simulink model "DFIG_BESS_In_power_LFnetwork_5bus"  (R2017b)
settings: Solver=ode23tb  StartTime=0.0  StopTime=7.5  MaxStep=0.04  RelTol=1e-3  EnableMultiTasking=on
values from neighbouring files (symbols this model uses):
  beta = beta (k)    [Parameter_2M_DFIG_BESS.m]
  Cbus = 80e-3    (= 0.08)    [Parameter_2M_DFIG_BESS.m]
  Cbus_bess = 15e-3    (= 0.015)    [Parameter_2M_DFIG_BESS.m]
  Cfilter = 80e-3    (= 0.08)    [Parameter_2M_DFIG_BESS.m]
  cp_opt_abs = abs(max(Cp))    [Parameter_2M_DFIG_BESS.m]
  D = 0.1    [Parameter_2M_DFIG_BESS.m]
  f = 60    [Parameter_2M_DFIG_BESS.m]
  Fs = 1.5    [Parameter_2M_DFIG_BESS.m]
  fsw = 4e3    (= 4000)    [Parameter_2M_DFIG_BESS.m]
  J = 90    [Parameter_2M_DFIG_BESS.m]
  ki_id = (wni^2)*Lr*sigma    (= 491.599501999)    [Parameter_2M_DFIG_BESS.m]
  ki_idg = (wnig^2)*Lg    (= 68.6450725305)    [Parameter_2M_DFIG_BESS.m]
  ki_iq = ki_id    (= 491.599501999)    [Parameter_2M_DFIG_BESS.m]
  ki_iqg = ki_idg    (= 68.6450725305)    [Parameter_2M_DFIG_BESS.m]
  ki_v = -300000    [Parameter_2M_DFIG_BESS.m]
  kp_id = (2*wni*sigma*Lr)-Rr    (= 0.5771)    [Parameter_2M_DFIG_BESS.m]
  kp_idg = (2*wnig*Lg)-Rg    (= 0.364153420404)    [Parameter_2M_DFIG_BESS.m]
  kp_iq = kp_id    (= 0.5771)    [Parameter_2M_DFIG_BESS.m]
  kp_iqg = kp_idg    (= 0.364153420404)    [Parameter_2M_DFIG_BESS.m]
  kp_v = -1000    [Parameter_2M_DFIG_BESS.m]
  Kpg = 1/(1.5*Vs*sqrt(2/3))    [Parameter_2M_DFIG_BESS.m]
  Kqg = -Kpg    [Parameter_2M_DFIG_BESS.m]
  lambda_opt = abs(lambda(posicion))    [Parameter_2M_DFIG_BESS.m]
  Lfilter = 483e-6    (= 0.000483)    [Parameter_2M_DFIG_BESS.m]
  Lg = 483e-6    (= 0.000483)    [Parameter_2M_DFIG_BESS.m]
  Lm = 2.5e-3    (= 0.0025)    [Parameter_2M_DFIG_BESS.m]
  Lr = Lm + Lsr    (= 0.002587)    [Parameter_2M_DFIG_BESS.m]
  Ls = Lm + Lsi    (= 0.002587)    [Parameter_2M_DFIG_BESS.m]
  Lsi = 87e-6    (= 8.7e-05)    [Parameter_2M_DFIG_BESS.m]
  n = 1800    [Parameter_2M_DFIG_BESS.m]
  N = 100    [Parameter_2M_DFIG_BESS.m]
  p = 2    [Parameter_2M_DFIG_BESS.m]
  Ps = 2e6    (= 2000000)    [Parameter_2M_DFIG_BESS.m]
  Radio = 44    [Parameter_2M_DFIG_BESS.m]
  Rfilter = 20e-3    (= 0.02)    [Parameter_2M_DFIG_BESS.m]
  ro = 1.225    [Parameter_2M_DFIG_BESS.m]
  Rr = 2.9e-3    (= 0.0029)    [Parameter_2M_DFIG_BESS.m]
  Rs = 2.6e-3    (= 0.0026)    [Parameter_2M_DFIG_BESS.m]
  sigma = 1- Lm^2/(Ls*Lr)    (= 0.0661284179513)    [Parameter_2M_DFIG_BESS.m]
  Ts = 1/fsw/f    (= 4.16666666667e-06)    [Parameter_2M_DFIG_BESS.m]
  Vbus_ref = 1200    [Parameter_2M_DFIG_BESS.m]
  Vdc_bat_ref = 1300    [Parameter_2M_DFIG_BESS.m]
  Vs = 690    [Parameter_2M_DFIG_BESS.m]
undefined symbols (not defined in the file or in its folder): D1, D11, Delta, DiscIntNeverNeededParam, Ion, Lithium, sigbuilder_block
libraries: powerlib x83, powerlib_meascontrol x28, sps_avr x2, electricdrivelib x1, peGeneralControl x1
(part 2 of 3)

== system DFIG_BESS_In_power_LFnetwork_5bus/Load N°2 6MW 2Mvar ==
  note: Consumer Load
  3-Phase Breaker : powerlib/Elements/Three-Phase Breaker  Commented=on  InitialState=open  SwitchA=on  SwitchB=on  SwitchC=on  SwitchTimes=[7]  External=off  BreakerResistance=0.001  SnubberResistance=1e6  SnubberCapacitance=inf  Measurements=None
      settings: AttributesFormatString=\n
  Load : powerlib/Measurements/Three-Phase V-I Measurement  VoltageMeasurement=no  SetLabelV=on  LabelV=Vabc_Load_B3  Vpu=off  VpuLL=off  CurrentMeasurement=no  SetLabelI=on  LabelI=Iabc_Load_B3  Ipu=off  Pbase=25e3  Vbase=480  OutputType=Magnitude  PhasorSimulation=off  PSBequivalent=0
  Main Load 10MW : powerlib/Elements/Three-Phase Parallel RLC Load  LConnTagsString=A|B|C  Configuration=Y (grounded)  NominalVoltage=33e+03  Vabc=[1e3 1e3 1e3]  Vabcp=[1e3 1e3 1e3]  NominalFrequency=60  UnbalancedPower=off  ActivePower=6e+06  InductivePower=2e+06  CapacitivePower=0  Pabc=[10e3 9e3 11e3]  QLabc=[100 90 110]  QCabc=[100 90 110]  Pabcp=[10e3 9e3 11e3]  QLabcp=[100 90 110]  QCabcp=[100 90 110]  Measurements=None  LoadType=constant Z
  Main Load 10M : powerlib/Elements/Three-Phase Parallel RLC Load  Commented=on  LConnTagsString=A|B|C  Configuration=Y (grounded)  NominalVoltage=33e+03  Vabc=[1e3 1e3 1e3]  Vabcp=[1e3 1e3 1e3]  NominalFrequency=60  UnbalancedPower=off  ActivePower=10e+06  InductivePower=0  CapacitivePower=0  Pabc=[10e3 9e3 11e3]  QLabc=[100 90 110]  QCabc=[100 90 110]  Pabcp=[10e3 9e3 11e3]  QLabcp=[100 90 110]  QCabcp=[100 90 110]  Measurements=None  LoadType=constant Z
  PLL (3ph)1 : powerlib_meascontrol/PLL/PLL (3ph)  Commented=on  Fmin=45  Par_Init=[0, f]  ParK=[180, 3200, 1]  TcD=1e-4  MaxRateChangeFreq=12  FilterCutOffFreq=25  Ts=0  AGC=on
  "Power (3ph, Instantaneous)1" : powerlib_meascontrol/Measurements/Power (3ph, Instantaneous)  Commented=on
      settings: SourceProductName=Simscape Power Systems
  Scope : Scope  Commented=on
  Vbus vcc1 : From  Commented=on  GotoTag=Iabc_Load_B3  TagVisibility=global
  Vbus vcc2 : From  Commented=on  GotoTag=Vabc_Load_B3  TagVisibility=global
  A : PMIOPort  Port=1  Side=Right
  B : PMIOPort  Port=2  Side=Right
  C : PMIOPort  Port=3  Side=Right
  wires:
  Vbus vcc1/1 -> "Power (3ph, Instantaneous)1"/2
  Vbus vcc2/1 -> PLL (3ph)1/1, "Power (3ph, Instantaneous)1"/1
  "Power (3ph, Instantaneous)1"/1 -> Scope/1
  connections:
  3-Phase Breaker/LConn2 -- Load/RConn2 -- Main Load 10MW/LConn2
  3-Phase Breaker/LConn3 -- Load/RConn3 -- Main Load 10MW/LConn3
  3-Phase Breaker/LConn1 -- Load/RConn1 -- Main Load 10MW/LConn1
  3-Phase Breaker/RConn2 -- Main Load 10M/LConn2
  3-Phase Breaker/RConn1 -- Main Load 10M/LConn1
  3-Phase Breaker/RConn3 -- Main Load 10M/LConn3
  A/RConn1 -- Load/LConn1
  B/RConn1 -- Load/LConn2
  C/RConn1 -- Load/LConn3

== system DFIG_BESS_In_power_LFnetwork_5bus/Load N°3 24MW 5Mvar ==
  note: Consumer Load
  " Load" : powerlib/Elements/Three-Phase Parallel RLC Load  Commented=on  LConnTagsString=A|B|C  Configuration=Y (grounded)  NominalVoltage=33e+03  Vabc=[1e3 1e3 1e3]  Vabcp=[1e3 1e3 1e3]  NominalFrequency=60  UnbalancedPower=off  ActivePower=5e+06  InductivePower=0  CapacitivePower=0  Pabc=[10e3 9e3 11e3]  QLabc=[100 90 110]  QCabc=[100 90 110]  Pabcp=[10e3 9e3 11e3]  QLabcp=[100 90 110]  QCabcp=[100 90 110]  Measurements=None  LoadType=constant Z
  3-Phase Breaker : powerlib/Elements/Three-Phase Breaker  Commented=on  InitialState=open  SwitchA=on  SwitchB=on  SwitchC=on  SwitchTimes=[7]  External=off  BreakerResistance=0.001  SnubberResistance=1e6  SnubberCapacitance=inf  Measurements=None
      settings: AttributesFormatString=\n
  Load : powerlib/Measurements/Three-Phase V-I Measurement  VoltageMeasurement=no  SetLabelV=on  LabelV=Vabc_Load_B4  Vpu=off  VpuLL=off  CurrentMeasurement=no  SetLabelI=on  LabelI=Iabc_Load_B4  Ipu=off  Pbase=25e3  Vbase=480  OutputType=Magnitude  PhasorSimulation=off  PSBequivalent=0
  Main Load 10MW : powerlib/Elements/Three-Phase Parallel RLC Load  LConnTagsString=A|B|C  Configuration=Y (grounded)  NominalVoltage=33e+03  Vabc=[1e3 1e3 1e3]  Vabcp=[1e3 1e3 1e3]  NominalFrequency=60  UnbalancedPower=off  ActivePower=24e+06  InductivePower=5e+06  CapacitivePower=0  Pabc=[10e3 9e3 11e3]  QLabc=[100 90 110]  QCabc=[100 90 110]  Pabcp=[10e3 9e3 11e3]  QLabcp=[100 90 110]  QCabcp=[100 90 110]  Measurements=None  LoadType=constant Z
  PLL (3ph)1 : powerlib_meascontrol/PLL/PLL (3ph)  Commented=on  Fmin=45  Par_Init=[0, f]  ParK=[180, 3200, 1]  TcD=1e-4  MaxRateChangeFreq=12  FilterCutOffFreq=25  Ts=0  AGC=on
  "Power (3ph, Instantaneous)1" : powerlib_meascontrol/Measurements/Power (3ph, Instantaneous)  Commented=on
      settings: SourceProductName=Simscape Power Systems
  Scope : Scope  Commented=on
  Vbus vcc1 : From  Commented=on  GotoTag=Iabc_Load_B4  TagVisibility=global
  Vbus vcc2 : From  Commented=on  GotoTag=Vabc_Load_B4  TagVisibility=global
  A : PMIOPort  Port=1  Side=Right
  B : PMIOPort  Port=2  Side=Right
  C : PMIOPort  Port=3  Side=Right
  wires:
  "Power (3ph, Instantaneous)1"/1 -> Scope/1
  Vbus vcc2/1 -> "Power (3ph, Instantaneous)1"/1, PLL (3ph)1/1
  Vbus vcc1/1 -> "Power (3ph, Instantaneous)1"/2
  connections:
  C/RConn1 -- Load/LConn3
  B/RConn1 -- Load/LConn2
  A/RConn1 -- Load/LConn1
  3-Phase Breaker/RConn3 -- " Load"/LConn3
  3-Phase Breaker/RConn1 -- " Load"/LConn1
  3-Phase Breaker/RConn2 -- " Load"/LConn2
  Load/RConn1 -- 3-Phase Breaker/LConn1 -- Main Load 10MW/LConn1
  Load/RConn3 -- 3-Phase Breaker/LConn3 -- Main Load 10MW/LConn3
  Load/RConn2 -- 3-Phase Breaker/LConn2 -- Main Load 10MW/LConn2

== system DFIG_BESS_In_power_LFnetwork_5bus/Load N°4 12MW 3Mvar Load N°5 5MW 2Mvar ==
  note: Load 5
  note: Load 4
  " Load" : powerlib/Elements/Three-Phase Parallel RLC Load  Commented=on  LConnTagsString=A|B|C  Configuration=Y (grounded)  NominalVoltage=33e+03  Vabc=[1e3 1e3 1e3]  Vabcp=[1e3 1e3 1e3]  NominalFrequency=60  UnbalancedPower=off  ActivePower=5e+06  InductivePower=2e+06  CapacitivePower=0  Pabc=[10e3 9e3 11e3]  QLabc=[100 90 110]  QCabc=[100 90 110]  Pabcp=[10e3 9e3 11e3]  QLabcp=[100 90 110]  QCabcp=[100 90 110]  Measurements=None  LoadType=constant Z
  3-Phase Breaker : powerlib/Elements/Three-Phase Breaker  Commented=on  InitialState=open  SwitchA=on  SwitchB=on  SwitchC=on  SwitchTimes=[5]  External=off  BreakerResistance=0.001  SnubberResistance=1e6  SnubberCapacitance=inf  Measurements=None
      settings: AttributesFormatString=\n
  Load : powerlib/Measurements/Three-Phase V-I Measurement  VoltageMeasurement=no  SetLabelV=on  LabelV=Vabc_Load_B4  Vpu=off  VpuLL=off  CurrentMeasurement=no  SetLabelI=on  LabelI=Iabc_Load_B4  Ipu=off  Pbase=25e3  Vbase=480  OutputType=Magnitude  PhasorSimulation=off  PSBequivalent=0
  Main Load 10MW : powerlib/Elements/Three-Phase Parallel RLC Load  LConnTagsString=A|B|C  Configuration=Y (grounded)  NominalVoltage=33e+03  Vabc=[1e3 1e3 1e3]  Vabcp=[1e3 1e3 1e3]  NominalFrequency=60  UnbalancedPower=off  ActivePower=12e+06  InductivePower=3e+06  CapacitivePower=0  Pabc=[10e3 9e3 11e3]  QLabc=[100 90 110]  QCabc=[100 90 110]  Pabcp=[10e3 9e3 11e3]  QLabcp=[100 90 110]  QCabcp=[100 90 110]  Measurements=None  LoadType=constant Z
  PLL (3ph)1 : powerlib_meascontrol/PLL/PLL (3ph)  Commented=on  Fmin=45  Par_Init=[0, f]  ParK=[180, 3200, 1]  TcD=1e-4  MaxRateChangeFreq=12  FilterCutOffFreq=25  Ts=0  AGC=on
  "Power (3ph, Instantaneous)1" : powerlib_meascontrol/Measurements/Power (3ph, Instantaneous)  Commented=on
      settings: SourceProductName=Simscape Power Systems
  Scope : Scope  Commented=on
  Vbus vcc1 : From  Commented=on  GotoTag=Iabc_Load_B4  TagVisibility=global
  Vbus vcc2 : From  Commented=on  GotoTag=Vabc_Load_B4  TagVisibility=global
  A : PMIOPort  Port=1  Side=Right
  B : PMIOPort  Port=2  Side=Right
  C : PMIOPort  Port=3  Side=Right
  wires:
  Vbus vcc1/1 -> "Power (3ph, Instantaneous)1"/2
  Vbus vcc2/1 -> PLL (3ph)1/1, "Power (3ph, Instantaneous)1"/1
  "Power (3ph, Instantaneous)1"/1 -> Scope/1
  connections:
  Main Load 10MW/LConn2 -- 3-Phase Breaker/LConn2 -- Load/RConn2
  Main Load 10MW/LConn3 -- 3-Phase Breaker/LConn3 -- Load/RConn3
  Main Load 10MW/LConn1 -- 3-Phase Breaker/LConn1 -- Load/RConn1
  3-Phase Breaker/RConn2 -- " Load"/LConn2
  3-Phase Breaker/RConn1 -- " Load"/LConn1
  3-Phase Breaker/RConn3 -- " Load"/LConn3
  A/RConn1 -- Load/LConn1
  B/RConn1 -- Load/LConn2
  C/RConn1 -- Load/LConn3

== system DFIG_BESS_In_power_LFnetwork_5bus/Power ==
  "Power (3ph, Instantaneous)1" : powerlib_meascontrol/Measurements/Power (3ph, Instantaneous)
      settings: SourceProductName=Simscape Power Systems
  P : Outport
  wires:
  [Vabc_B1] -> "Power (3ph, Instantaneous)1"/1
  [Iabc_B1] -> "Power (3ph, Instantaneous)1"/2
  "Power (3ph, Instantaneous)1"/1 -> P/1

== system DFIG_BESS_In_power_LFnetwork_5bus/Power1 ==
  "Power (3ph, Instantaneous)1" : powerlib_meascontrol/Measurements/Power (3ph, Instantaneous)
      settings: SourceProductName=Simscape Power Systems
  P : Outport
  wires:
  "Power (3ph, Instantaneous)1"/1 -> P/1
  [Iabc_G] -> "Power (3ph, Instantaneous)1"/2
  [Vabc_G] -> "Power (3ph, Instantaneous)1"/1

== system DFIG_BESS_In_power_LFnetwork_5bus/Power2 ==
  "Power (3ph, Instantaneous)1" : powerlib_meascontrol/Measurements/Power (3ph, Instantaneous)
      settings: SourceProductName=Simscape Power Systems
  P : Outport
  wires:
  "Power (3ph, Instantaneous)1"/1 -> P/1
  [I_ac_g] -> "Power (3ph, Instantaneous)1"/2
  [V_ac_g] -> "Power (3ph, Instantaneous)1"/1

== system DFIG_BESS_In_power_LFnetwork_5bus/Power3 ==
  "Power (3ph, Instantaneous)1" : powerlib_meascontrol/Measurements/Power (3ph, Instantaneous)
      settings: SourceProductName=Simscape Power Systems
  P : Outport
  wires:
  [V_ac_bess_HV] -> "Power (3ph, Instantaneous)1"/1
  [I_ac_bess_HV] -> "Power (3ph, Instantaneous)1"/2
  "Power (3ph, Instantaneous)1"/1 -> P/1

== system DFIG_BESS_In_power_LFnetwork_5bus/Power4 ==
  "Power (3ph, Instantaneous)1" : powerlib_meascontrol/Measurements/Power (3ph, Instantaneous)
      settings: SourceProductName=Simscape Power Systems
  P : Outport
  wires:
  [V_ac_g_Total] -> "Power (3ph, Instantaneous)1"/1
  [I_ac_g_Total] -> "Power (3ph, Instantaneous)1"/2
  "Power (3ph, Instantaneous)1"/1 -> P/1

== system DFIG_BESS_In_power_LFnetwork_5bus/Subsystem1 ==
  " Iabc (pu)" : Scope  NumInputPorts=2
  " Load 3 MW 2 Mvar" : powerlib/Elements/Three-Phase Parallel RLC Load  LConnTagsString=A|B|C  Configuration=Y (grounded)  NominalVoltage=(13800)*0.98  Vabc=[1e3 1e3 1e3]  Vabcp=[1e3 1e3 1e3]  NominalFrequency=60  UnbalancedPower=off  ActivePower=3000000  InductivePower=2000000  CapacitivePower=0  Pabc=[10e3 9e3 11e3]  QLabc=[100 90 110]  QCabc=[100 90 110]  Pabcp=[10e3 9e3 11e3]  QLabcp=[100 90 110]  QCabcp=[100 90 110]  Measurements=None  LoadType=constant PQ
  " Speed (pu)" : Scope
  Bus Selector : BusSelector  OutputSignals="Stator current,Output active power   Peo (pu)"
  Bus Selector1 : BusSelector  OutputSignals="dq0 components.Stator voltage  vq (pu),dq0 components.Stator voltage  vd (pu),Mechanical.Rotor speed  wm  (pu),Mechanical.Rotor speed deviation  dw (pu),Output active power   Peo (pu)"
  Display3 : Display
  Excitation System : sps_avr/Excitation System  tr=20e-3  reg=[ 300, 0.001 ]  exc=[ 1, 0 ]  tgr=[ 0, 0 ]  damp=[ 0.001, 0.1 ]  sat=[ 0, 0 ]  lim=[ -11.5, 11.5, 0 ]  v0=[1,1.29071]
      settings: SourceProductName=Simscape Power Systems  SourceProductBaseCode=PS
  Ground : Ground
  HTG : powerlib/Machines/Hydraulic Turbine and Governor  sm="[ 10/3  0.07 ]"  gate="[  0.01  0.97518  -0.1  0.1 ]"  reg="[  0.05  1.163  0.105  0  0.01  ]"  hyd="[  0  2.67  ]"  dref=0  po=1
      settings: SourceProductName=Simscape Power Systems  SourceProductBaseCode=PS
  Pref : Constant
  "Synchronous Machine " : powerlib/Machines/Synchronous Machine pu Standard  PresetModel=No  MechanicalLoad=Mechanical power Pm  ShowDetailedParameters=on  RotorType=Salient-pole  Units=per unit standard parameters  MeasurementBus=off  NominalParameters="[50e+06  13800   f ]"  Reactances1=[ 31 32 33 34 35 36 37 ]  Reactances2=[ 1.305, 0.296, 0.252, 0.474, 0.243, 0.18 ]  dAxisTimeConstants=Short-circuit  qAxisTimeConstants=Open-circuit  TimeConstants1=[]  TimeConstants2=[]  TimeConstants3=[]  TimeConstants4=[]  TimeConstants5=[ 1.01, 0.053, 0.1 ]  TimeConstants6=[]  TimeConstants7=[]  TimeConstants8=[]  StatorResistance=2.8544e-3  Mechanical=[ 3.2 0 2]  PolePairs=2  InitialConditions=[0 -94.2826 0.750185 0.750185 0.750185 -24.943 -144.943 95.057 1.29071]  SetSaturation=off  Saturation=[0.6404,0.7127,0.8441,0.9214,0.9956,1.082,1.19,1.316,1.457;0.7,0.7698,0.8872,0.9466,0.9969,1.046,1.1,1.151,1.201]  LoadFlowParameters=[1 150000000 0 0]  TsPowergui=0  TsBlock=-1  IterativeModel=Trapezoidal non iterative  IterativeDiscreteModel=Trapezoidal non iterative  BusType=PQ  Pref=50e+06  Qref=0  Qmin=-Inf  Qmax=Inf  PLF=0  QLF=0
      settings: AttributesFormatString=\n\n  SourceProductName=Simscape Power Systems
  Terminator5 : Terminator
  Vf (pu) : Scope
  Vref : Constant
  wref : Constant
  Va : PMIOPort  Port=1  Side=Left
  Vb : PMIOPort  Port=2  Side=Left
  Vc : PMIOPort  Port=3  Side=Left
  wires:
  HTG/1 -> Display3/1, "Synchronous Machine "/1
  Bus Selector/2 -> " Iabc (pu)"/2  "<Output active power   Peo (pu)>"
  "Synchronous Machine "/1 -> Bus Selector1/1, Bus Selector/1
  Vref/1 -> Excitation System/1
  wref/1 -> HTG/1
  Pref/1 -> HTG/2
  Bus Selector1/4 -> HTG/5  "<Rotor speed deviation  dw (pu)>"
  Excitation System/1 -> "Synchronous Machine "/2, Vf (pu)/1
  Bus Selector1/1 -> Excitation System/3  "<Stator voltage  vq (pu)>"
  Ground/1 -> Excitation System/4
  Bus Selector1/2 -> Excitation System/2  "<Stator voltage  vd (pu)>"
  Bus Selector/1 -> " Iabc (pu)"/1  "<Stator current>"
  Bus Selector1/3 -> " Speed (pu)"/1, HTG/3  "<Rotor speed  wm  (pu)>"
  HTG/2 -> Terminator5/1
  Bus Selector1/5 -> HTG/4  "<Output active power   Peo (pu)>"
  connections:
  " Load 3 MW 2 Mvar"/LConn3 -- "Synchronous Machine "/RConn3 -- Vc/RConn1
  " Load 3 MW 2 Mvar"/LConn2 -- Vb/RConn1 -- "Synchronous Machine "/RConn2
  " Load 3 MW 2 Mvar"/LConn1 -- "Synchronous Machine "/RConn1 -- Va/RConn1

== system DFIG_BESS_In_power_LFnetwork_5bus/Subsystem2 ==
  " Iabc (pu)" : Scope  NumInputPorts=2
  " Load 3 MW 2 Mvar" : powerlib/Elements/Three-Phase Parallel RLC Load  LConnTagsString=A|B|C  Configuration=Y (grounded)  NominalVoltage=(13800)*0.98  Vabc=[1e3 1e3 1e3]  Vabcp=[1e3 1e3 1e3]  NominalFrequency=60  UnbalancedPower=off  ActivePower=3000000  InductivePower=2000000  CapacitivePower=0  Pabc=[10e3 9e3 11e3]  QLabc=[100 90 110]  QCabc=[100 90 110]  Pabcp=[10e3 9e3 11e3]  QLabcp=[100 90 110]  QCabcp=[100 90 110]  Measurements=None  LoadType=constant PQ
  " Speed (pu)" : Scope
  Bus Selector : BusSelector  OutputSignals="Stator current,Output active power   Peo (pu)"
  Bus Selector1 : BusSelector  OutputSignals="dq0 components.Stator voltage  vq (pu),dq0 components.Stator voltage  vd (pu),Mechanical.Rotor speed  wm  (pu),Mechanical.Rotor speed deviation  dw (pu),Output active power   Peo (pu)"
  Display3 : Display
  Excitation System : sps_avr/Excitation System  tr=20e-3  reg=[ 300, 0.001 ]  exc=[ 1, 0 ]  tgr=[ 0, 0 ]  damp=[ 0.001, 0.1 ]  sat=[ 0, 0 ]  lim=[ -11.5, 11.5, 0 ]  v0=[1,1.29071]
      settings: SourceProductName=Simscape Power Systems  SourceProductBaseCode=PS
  Ground : Ground
  HTG : powerlib/Machines/Hydraulic Turbine and Governor  sm="[ 10/3  0.07 ]"  gate="[  0.01  0.97518  -0.1  0.1 ]"  reg="[  0.05  1.163  0.105  0  0.01  ]"  hyd="[  0  2.67  ]"  dref=0  po=1
      settings: SourceProductName=Simscape Power Systems  SourceProductBaseCode=PS
  Pref : Constant
  "Synchronous Machine " : powerlib/Machines/Synchronous Machine pu Standard  PresetModel=No  MechanicalLoad=Mechanical power Pm  ShowDetailedParameters=on  RotorType=Salient-pole  Units=per unit standard parameters  MeasurementBus=off  NominalParameters="[30e+06  13800   f ]"  Reactances1=[ 31 32 33 34 35 36 37 ]  Reactances2=[ 1.305, 0.296, 0.252, 0.474, 0.243, 0.18 ]  dAxisTimeConstants=Short-circuit  qAxisTimeConstants=Open-circuit  TimeConstants1=[]  TimeConstants2=[]  TimeConstants3=[]  TimeConstants4=[]  TimeConstants5=[ 1.01, 0.053, 0.1 ]  TimeConstants6=[]  TimeConstants7=[]  TimeConstants8=[]  StatorResistance=2.8544e-3  Mechanical=[ 3.2 0 2]  PolePairs=2  InitialConditions=[0 -94.2826 0.750185 0.750185 0.750185 -24.943 -144.943 95.057 1.29071]  SetSaturation=off  Saturation=[0.6404,0.7127,0.8441,0.9214,0.9956,1.082,1.19,1.316,1.457;0.7,0.7698,0.8872,0.9466,0.9969,1.046,1.1,1.151,1.201]  LoadFlowParameters=[1 150000000 0 0]  TsPowergui=0  TsBlock=-1  IterativeModel=Trapezoidal non iterative  IterativeDiscreteModel=Trapezoidal non iterative  BusType=PQ  Pref=30e+06  Qref=0  Qmin=-Inf  Qmax=Inf  PLF=0  QLF=0
      settings: AttributesFormatString=\n\n  SourceProductName=Simscape Power Systems
  Terminator5 : Terminator
  Vf (pu) : Scope
  Vref : Constant
  wref : Constant
  Va : PMIOPort  Port=1  Side=Left
  Vb : PMIOPort  Port=2  Side=Left
  Vc : PMIOPort  Port=3  Side=Left
  wires:
  Bus Selector1/5 -> HTG/4  "<Output active power   Peo (pu)>"
  HTG/2 -> Terminator5/1
  Bus Selector1/3 -> HTG/3, " Speed (pu)"/1  "<Rotor speed  wm  (pu)>"
  Bus Selector/1 -> " Iabc (pu)"/1  "<Stator current>"
  Bus Selector1/2 -> Excitation System/2  "<Stator voltage  vd (pu)>"
  Ground/1 -> Excitation System/4
  Bus Selector1/1 -> Excitation System/3  "<Stator voltage  vq (pu)>"
  Excitation System/1 -> Vf (pu)/1, "Synchronous Machine "/2
  Bus Selector1/4 -> HTG/5  "<Rotor speed deviation  dw (pu)>"
  Pref/1 -> HTG/2
  wref/1 -> HTG/1
  Vref/1 -> Excitation System/1
  "Synchronous Machine "/1 -> Bus Selector/1, Bus Selector1/1
  Bus Selector/2 -> " Iabc (pu)"/2  "<Output active power   Peo (pu)>"
  HTG/1 -> "Synchronous Machine "/1, Display3/1
  connections:
  "Synchronous Machine "/RConn1 -- " Load 3 MW 2 Mvar"/LConn1 -- Va/RConn1
  Vb/RConn1 -- " Load 3 MW 2 Mvar"/LConn2 -- "Synchronous Machine "/RConn2
  "Synchronous Machine "/RConn3 -- " Load 3 MW 2 Mvar"/LConn3 -- Vc/RConn1

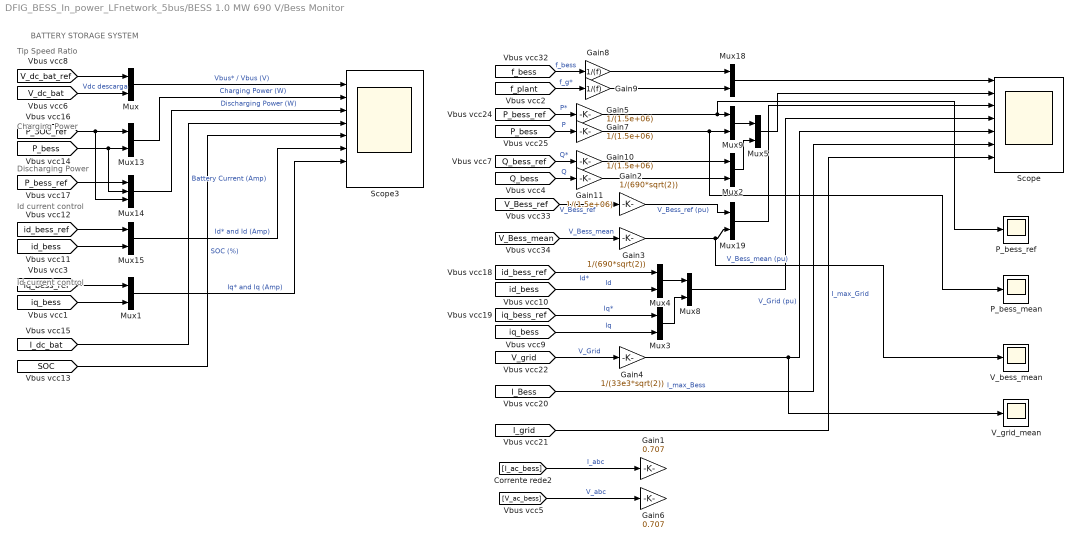
== system DFIG_BESS_In_power_LFnetwork_5bus/BESS 1.0 MW 690 V/Bess Monitor ==
  note: BATTERY STORAGE SYSTEM
  note: Tip Speed Ratio
  note: Charging Power
  note: Discharging Power
  note: Id current control
  note: Id current control
  Gain1 : Gain  Gain=0.707
  Gain{5,7,10..11} (4 alike) : Gain  Gain=1/(1.5e+06)
  Gain2 : Gain  Gain=1/(690*sqrt(2))
  Gain3 : Gain  Gain=1/(690*sqrt(2))
  Gain4 : Gain  Gain=1/(33e3*sqrt(2))
  Gain6 : Gain  Gain=0.707
  Gain8 : Gain  Gain=1/(f)
  Gain9 : Gain  Gain=1/(f)
  Mux{,1..5,8..9,13,15,18..19} (12 alike) : Mux  Inputs=2
  Mux14 : Mux  Inputs=3
  P_bess_mean : Scope
  P_bess_ref : Scope
  Scope : Scope  NumInputPorts=8
  Scope3 : Scope  NumInputPorts=8
  V_bess_mean : Scope
  V_grid_mean : Scope
  wires:
  [P_bess_ref] -> Mux14/1
  Mux13/1 -> Scope3/2  "Charging Power (W)"
  [P_SOC_ref] -> Mux14/3, Mux13/1
  [P_bess] -> Mux14/2, Mux13/2
  [id_bess_ref] -> Mux15/1
  [V_dc_bat_ref] -> Mux/1
  Mux/1 -> Scope3/1  "Vbus* / Vbus (V)"
  [id_bess] -> Mux15/2
  Mux14/1 -> Scope3/3  "Discharging Power (W)"
  [SOC] -> Scope3/5  "SOC (%)"
  [I_dc_bat] -> Scope3/4  "Battery Current (Amp)"
  Mux15/1 -> Scope3/6  "Id* and Id (Amp)"
  [V_dc_bat] -> Mux/2  "Vdc descarga"
  [iq_bess] -> Mux1/2
  [iq_bess_ref] -> Mux1/1
  Mux1/1 -> Scope3/7  "Iq* and Iq (Amp)"
  [Q_bess_ref] -> Gain10/1  "Q*"
  [iq_bess_ref] -> Mux3/1  "Iq*"
  [id_bess] -> Mux4/2  "Id"
  [iq_bess] -> Mux3/2  "Iq"
  [id_bess_ref] -> Mux4/1  "Id*"
  Mux4/1 -> Mux8/1
  Mux3/1 -> Mux8/2
  [P_bess_ref] -> Gain5/1  "P*"
  [f_bess] -> Gain8/1  "f_bess"
  [f_plant] -> Gain9/1  "f_g*"
  Mux18/1 -> Scope/1
  [V_Bess_ref] -> Gain2/1  "V_Bess_ref"
  [V_Bess_mean] -> Gain3/1  "V_Bess_mean"
  [V_ac_bess] -> Gain6/1  "V_abc"
  [I_ac_bess] -> Gain1/1  "I_abc"
  [V_grid] -> Gain4/1  "V_Grid"
  [P_bess] -> Gain7/1  "P"
  [Q_bess] -> Gain11/1  "Q"
  Gain2/1 -> Mux19/1  "V_Bess_ref (pu)"
  Gain3/1 -> V_bess_mean/1, Mux19/2  "V_Bess_mean (pu)"
  Gain4/1 -> V_grid_mean/1, Scope/5  "V_Grid (pu)"
  [I_Bess] -> Scope/6  "I_max_Bess"
  [I_grid] -> Scope/7  "I_max_Grid"
  Mux19/1 -> Scope/3
  Mux8/1 -> Scope/4
  Gain5/1 -> P_bess_ref/1, Mux9/1
  Gain7/1 -> P_bess_mean/1, Mux9/2
  Gain8/1 -> Mux18/1
  Gain9/1 -> Mux18/2
  Mux9/1 -> Mux5/1
  Mux2/1 -> Mux5/2
  Mux5/1 -> Scope/2
  Gain10/1 -> Mux2/1
  Gain11/1 -> Mux2/2

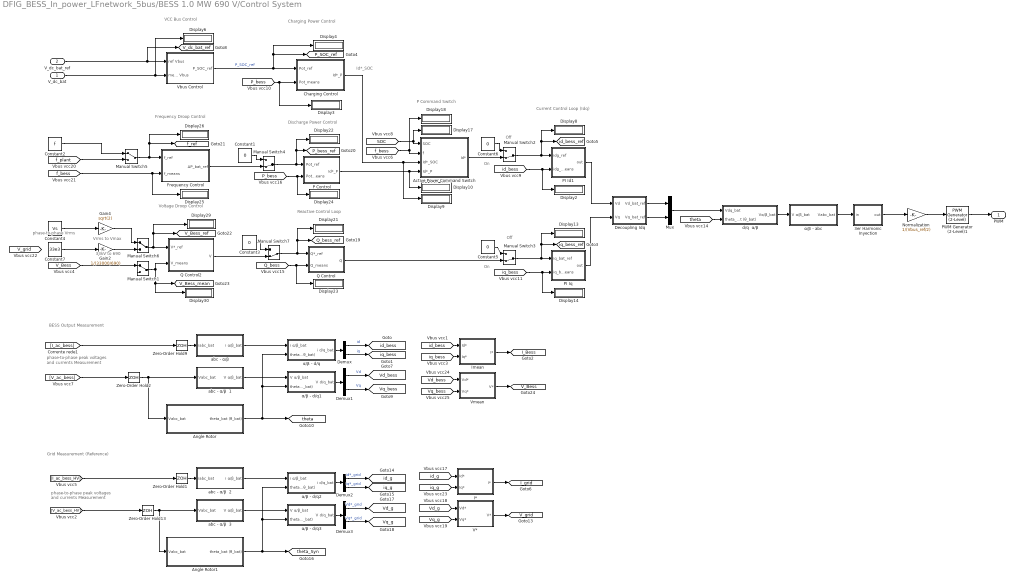
== system DFIG_BESS_In_power_LFnetwork_5bus/BESS 1.0 MW 690 V/Control System ==
  note: BESS Output Measurement
  note: Id*_SOC
  note: Grid Measurement (Reference)
  note: Current Control Loop (Idq)
  note: Discharge Power Control
  note: Frequency Droop Control
  note: VCC Bus Control
  note: Charging Power Control
  note: P Command Switch
  note: On
  note: Off
  note: On
  note: Off
  note: phase-to-phase peak voltages
      | and currents Measurement
  note: phase-to-phase peak voltages
      | and currents Measurement
  note: 33kV to 690
  note: Voltage Droop Control
  note: Reactive Control Loop
  note: Vrms to Vmax
  note: phase-to-phase Vrms
  V_dc_bat : Inport
  V_dc_bat_ref : Inport  Port=2
  " Angle Rotor" : Subsystem
  " Angle Rotor1" : Subsystem
  3er Harmonic Inyection : Subsystem
  Active Power Command Switch : Subsystem
  Charging Control : Subsystem
  Constant{1,3,5..6} (4 alike) : Constant  Value=0
  Constant2 : Constant  Value=f
  Constant4 : Constant  Value=Vs
  Constant7 : Constant  Value=33e3
  Decoupling Idq : Subsystem
  Demux{,1..3} (4 alike) : Demux  Outputs=2
  Display{2..4,6,8..10,13..14,17..18,21..26,29..30} (19 alike) : Display
  Frequency Control : Subsystem
  Gain2 : Gain  Gain=1/(33000/690)
  Gain4 : Gain  Gain=sqrt(2)
  I* : Subsystem
  Imean : Subsystem
  Manual Switch1 : ManualSwitch
  Manual Switch{2..4,7} (4 alike) : ManualSwitch  CurrentSetting=0
  Manual Switch5 : ManualSwitch
  Manual Switch6 : ManualSwitch
  Mux : Mux  Inputs=2
  Normalization : Gain  Gain=1/(Vbus_ref/2)
  P Control : Subsystem
  PI Id1 : Subsystem
  PI Iq : Subsystem
  PWM Generator (2-Level)1 : powerlib_meascontrol/Pulse & Signal Generators/PWM Generator (2-Level)  ModulatorType=Three-phase bridge (6 pulses)  ModulatorMode=Unsynchronized  Fc=fsw  Pc=0  nF=27  MinMax="[ -1  1 ]"  SamplingTechnique=Natural  ModulatingSignals=off  m=0.8  Freq=60  Phase=0  Ts=0  ShowCarrierOutport=off
      settings: SourceProductName=Simscape Power Systems
  Q Control : Subsystem
  Q Control2 : Subsystem
  V* : Subsystem
  Vbus Control : Subsystem
  Vmean : Subsystem
  Zero-Order Hold{1..2,9,13} (4 alike) : ZeroOrderHold  SampleTime=1/fsw
  "abc - α/β  " : Subsystem
  abc - α/β  1 : Subsystem
  abc - α/β  2 : Subsystem
  abc - α/β  3 : Subsystem
  "d/q  α/β " : Subsystem
  α/β - abc : Subsystem
  α/β - d/q : Subsystem
  α/β - d/q1 : Subsystem
  α/β - d/q2 : Subsystem
  α/β - d/q3 : Subsystem
  PWM : Outport
  tag scope: I_Bess=global, I_grid=global, P_SOC_ref=global, P_bess_ref=global, Q_bess_ref=global, V_Bess=global, V_Bess_mean=global, V_Bess_ref=global, V_dc_bat_ref=global, V_grid=global, Vd_bess=global, Vd_g=global, Vq_bess=global, Vq_g=global, f_ref=global, id_bess=global, id_bess_ref=global, id_g=global, iq_bess=global, iq_bess_ref=global, iq_g=global, theta=global, theta_Syn=global
  wires:
  PWM Generator (2-Level)1/1 -> PWM/1
  α/β - d/q/1(i d/q_bat) -> Demux/1
  Zero-Order Hold2/1 -> " Angle Rotor"/1(Vabc_bat), abc - α/β  1/1(Vabc_bat)
  α/β - abc/1(Vabc_bat) -> 3er Harmonic Inyection/1(in)
  Zero-Order Hold9/1 -> "abc - α/β  "/1(iabc_bat)
  "d/q  α/β "/1("Vα/β_bat ") -> α/β - abc/1(V α/β_bat)
  "abc - α/β  "/1(i α/β_bat) -> α/β - d/q/1(i α/β_bat)
  3er Harmonic Inyection/1(out) -> Normalization/1
  PI Id1/1(out) -> Decoupling Idq/1(Vd)
  PI Iq/1("out ") -> Decoupling Idq/2(Vq)
  Normalization/1 -> PWM Generator (2-Level)1/1
  V_dc_bat/1 -> Display6/1, Vbus Control/2("means Vbus ")
  [f_bess] -> Active Power Command Switch/2(f), Display18/1
  [SOC] -> Active Power Command Switch/1(SOC), Display17/1
  V_dc_bat_ref/1 -> [V_dc_bat_ref], Vbus Control/1("ref Vbus ")
  Vbus Control/1(P_SOC_ref) -> [P_SOC_ref], Display4/1, Charging Control/1("Pot_ref ")  "P_SOC_ref"
  [P_bess] -> Charging Control/2("Pot_means "), Display3/1
  Demux1/1 -> [Vd_bess]  "Vd"
  abc - α/β  1/1(V α/β_bat) -> α/β - d/q1/1(V α/β_bat)
  α/β - d/q1/1(V d/q_bat) -> Demux1/1
  Demux1/2 -> [Vq_bess]  "Vq"
  Mux/1 -> "d/q  α/β "/1(Vdq_bat)
  Decoupling Idq/1(" Vd_bat_ref") -> Mux/1
  Decoupling Idq/2(" Vq_bat_ref") -> Mux/2
  " Angle Rotor"/1(theta_bat (θ_bat)) -> α/β - d/q1/2(theta_bat (θ_bat)), α/β - d/q/2(theta_bat (θ_bat)), [theta]
  Demux/1 -> [id_bess]  "id"
  Demux/2 -> [iq_bess]  "iq"
  [theta] -> "d/q  α/β "/2(theta_bat (θ_bat))
  [id_bess] -> PI Id1/2(idg_means), Display2/1
  [iq_bess] -> Display14/1, PI Iq/2(iq_bat_means)
  Demux3/2 -> [Vq_g]  "Vq*_grid"
  Demux3/1 -> [Vd_g]  "Vd*_grid"
  abc - α/β  3/1(V α/β_bat) -> α/β - d/q3/1(V α/β_bat)
  abc - α/β  2/1(i α/β_bat) -> α/β - d/q2/1(i α/β_bat)
  " Angle Rotor1"/1(theta_bat (θ_bat)) -> α/β - d/q3/2(theta_bat (θ_bat)), α/β - d/q2/2(theta_bat (θ_bat)), [theta_Syn]
  Demux2/1 -> [id_g]  "id*_grid"
  Demux2/2 -> [iq_g]  "iq*_grid"
  α/β - d/q2/1(i d/q_bat) -> Demux2/1
  α/β - d/q3/1(V d/q_bat) -> Demux3/1
  [I_ac_bess_HV] -> Zero-Order Hold1/1
  [V_ac_bess_HV] -> Zero-Order Hold13/1
  Zero-Order Hold1/1 -> abc - α/β  2/1(iabc_bat)
  Zero-Order Hold13/1 -> " Angle Rotor1"/1(Vabc_bat), abc - α/β  3/1(Vabc_bat)
  [P_bess] -> Display24/1, P Control/2("Pot_means ")
  Manual Switch2/1 -> Display8/1, [id_bess_ref], PI Id1/1(idg_ref)
  Manual Switch3/1 -> Display13/1, [iq_bess_ref], PI Iq/1(iq_bat_ref)
  [f_bess] -> Display25/1, Frequency Control/2(f_means)
  Manual Switch4/1 -> [P_bess_ref], Display22/1, P Control/1("Pot_ref ")
  Frequency Control/1("ΔP_bat_ref ") -> Manual Switch4/2
  Constant1/1 -> Manual Switch4/1
  Manual Switch5/1 -> Display26/1, [f_ref], Frequency Control/1(f_ref)
  [Vq_g] -> V*/2(Vq*)
  [Vd_g] -> V*/1(Vd*)
  [Vd_bess] -> Vmean/1(Vd*)
  [Vq_bess] -> Vmean/2(Vq*)
  [f_plant] -> Manual Switch5/2
  Constant2/1 -> Manual Switch5/1
  Constant5/1 -> Manual Switch3/1
  V*/1("V* ") -> [V_grid]
  Vmean/1("V* ") -> [V_Bess]
  [I_ac_bess] -> Zero-Order Hold9/1
  [V_ac_bess] -> Zero-Order Hold2/1
  Active Power Command Switch/1(Id*) -> Manual Switch2/2
  Charging Control/1(Id*_P) -> Display9/1, Active Power Command Switch/3(Id*_SOC)
  P Control/1(Id*_P) -> Active Power Command Switch/4(Id*_P), Display10/1
  Imean/1("I* ") -> [I_Bess]
  [iq_bess] -> Imean/2(Iq*)
  [id_bess] -> Imean/1(Id*)
  I*/1("I* ") -> [I_grid]
  [id_g] -> I*/1(Id*)
  [iq_g] -> I*/2(Iq*)
  Constant6/1 -> Manual Switch2/1
  [V_Bess] -> Manual Switch1/1
  Manual Switch1/1 -> Q Control2/2(V_means), Display30/1, [V_Bess_mean]
  Q Control/1("Q ") -> Manual Switch3/2
  Constant3/1 -> Manual Switch7/1
  Gain4/1 -> Manual Switch6/1
  Constant4/1 -> Gain4/1
  Manual Switch7/1 -> [Q_bess_ref], Display21/1, Q Control/1(Q*_ref)
  Q Control2/1("V ") -> Manual Switch7/2
  Gain2/1 -> Manual Switch6/2
  Manual Switch6/1 -> Q Control2/1(V*_ref), Display29/1, [V_Bess_ref]
  [Q_bess] -> Display23/1, Q Control/2(Q_means)
  Constant7/1 -> Gain2/1

== system DFIG_BESS_In_power_LFnetwork_5bus/BESS 1.0 MW 690 V/Measurement of Power - Frequency ==
  FP : Fcn  Commented=on  Expr=cos(atan(u[1]/u[2]))
  Manual Switch3 : ManualSwitch  CurrentSetting=0
  Mux : Mux  Commented=on  Inputs=2
  PLL (3ph)1 : powerlib_meascontrol/PLL/PLL (3ph)  Fmin=45  Par_Init=[0, f]  ParK=[180, 3200, 1]  TcD=1e-4  MaxRateChangeFreq=12  FilterCutOffFreq=25  Ts=0  AGC=on
  "Power (3ph, Instantaneous)1" : powerlib_meascontrol/Measurements/Power (3ph, Instantaneous)
      settings: SourceProductName=Simscape Power Systems
  Scope : Scope  Commented=on
  F (Hz) : Outport
  P (W) : Outport  Port=2
  Q (VAR) : Outport  Port=3
  Angle (0) : Outport  Port=4
  tag scope: P_bess=global, Q_bess=global, f_bess=global, wt_mean=global
  wires:
  [V_ac_bess] -> "Power (3ph, Instantaneous)1"/1, PLL (3ph)1/1
  "Power (3ph, Instantaneous)1"/1 -> [P_bess], Mux/2, P (W)/1  "Pot"
  [I_ac_bess] -> "Power (3ph, Instantaneous)1"/2
  "Power (3ph, Instantaneous)1"/2 -> Mux/1, Q (VAR)/1, [Q_bess]
  PLL (3ph)1/2 -> Angle (0)/1, [wt_mean]
  Mux/1 -> FP/1
  FP/1 -> Scope/1
  [f_dfig_bess] -> Manual Switch3/1
  PLL (3ph)1/1 -> Manual Switch3/2
  Manual Switch3/1 -> F (Hz)/1, [f_bess]

== system DFIG_BESS_In_power_LFnetwork_5bus/BESS 1.0 MW 690 V/Subsystem1 ==
  In1 : Inport
  Bus Selector : BusSelector  OutputSignals=SOC (%),Current (A),Voltage (V)
  tag scope: I_dc_bat=global, SOC=global, V_dc_bat=global
  wires:
  Bus Selector/3 -> [V_dc_bat]  "<Voltage (V)>"
  Bus Selector/1 -> [SOC]  "<SOC (%)>"
  In1/1 -> Bus Selector/1
  Bus Selector/2 -> [I_dc_bat]  "<Current (A)>"

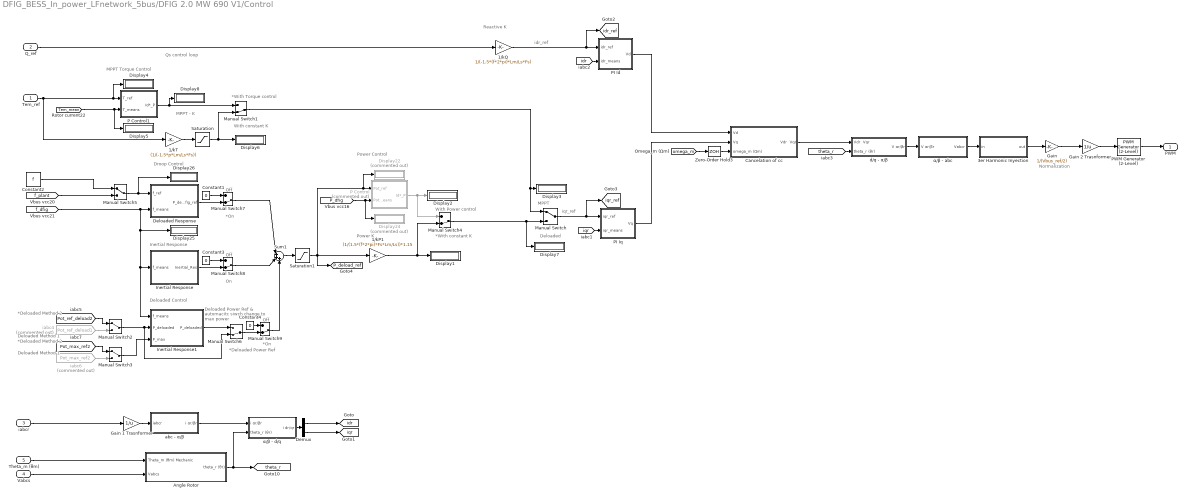
== system DFIG_BESS_In_power_LFnetwork_5bus/DFIG 2.0 MW 690 V1/Control ==
  note: Normalization
  note: iqr_ref
  note: idr_ref
  note: Qs control loop
  note: Reactive K
  note: MPPT - K
  note: Droop Control
  note: Power Control
  note: Power K
  note: MPPT
  note: Deloaded
  note: MPPT Torque Control
  note: Inertial Response
  note: Deloaded Control
  note: *Deloaded Power Ref
  note: Deloaded Power Ref &
      | automacitc siwch change
      | to max power
  note: *With constant K
  note: With Power control
  note: *With Torque control
  note: With constant K
  note: Deloaded Method 1
  note: Deloaded Method 1
  note: *Deloaded Method 2
  note: *Deloaded Method 2
  note: On
  note: *On
  note: *On
  note: Off
  note: Off
  note: Off
  Tem_ref : Inport
  Q_ref : Inport  Port=2
  iabcr : Inport  Port=3
  Vabcs : Inport  Port=4
  Theta_m (θm) : Inport  Port=5
  " Angle Rotor" : Subsystem
  1/kP1 : Gain  Gain=(1/(1.5*(f*2*pi)*Fs*Lm/Ls))*1.15
  1/kQ : Gain  Gain=1/(-1.5*(f*2*pi)*Lm/Ls*Fs)
  1/kT : Gain  Gain=(1/(-1.5*p*Lm/Ls*Fs))
  3er Harmonic Inyection : Subsystem
  Cancelation of cc : Subsystem
  Constant1 : Constant  Value=0
  Constant2 : Constant  Value=f
  Constant3 : Constant  Value=0
  Constant4 : Constant  Value=0
  Deloaded Response : Subsystem
  Demux : Demux  Outputs=2
  Display{1..8,25..26} (10 alike) : Display
  Display22 : Display  Commented=on
  Display24 : Display  Commented=on
  Gain : Gain  Gain=1/(Vbus_ref/2)
  Gain 1 Trasnformer : Gain  Gain=1/u
  Gain 2 Trasnformer : Gain  Gain=1/u
  Inertial Response : Subsystem
  Inertial Response1 : Subsystem
  Manual Switch{,2..3,5} (4 alike) : ManualSwitch
  Manual Switch{1,4,6..9} (6 alike) : ManualSwitch  CurrentSetting=0
  P Control : Subsystem  Commented=on
  P Control1 : Subsystem
  PI Id : Subsystem
  PI Iq : Subsystem
  PWM Generator (2-Level) : powerlib_meascontrol/Pulse & Signal Generators/PWM Generator (2-Level)  ModulatorType=Three-phase bridge (6 pulses)  ModulatorMode=Unsynchronized  Fc=fsw  Pc=0  nF=27  MinMax="[ -1  1 ]"  SamplingTechnique=Natural  ModulatingSignals=off  m=0.8  Freq=60  Phase=0  Ts=0  ShowCarrierOutport=off
      settings: SourceProductName=Simscape Power Systems
  Saturation : Saturate  UpperLimit=3500  LowerLimit=0
  Saturation1 : Saturate  UpperLimit=2.5e+06  LowerLimit=0
  Sum1 : Sum  Inputs=|+++
  Zero-Order Hold3 : ZeroOrderHold  SampleTime=1/fsw
  "abc - α/β " : Subsystem
  d/q - α/β : Subsystem
  iabc4 : From  Commented=on  GotoTag=Pot_ref_deload1  TagVisibility=global
  iabc6 : From  Commented=on  GotoTag=Pot_max_ref2  TagVisibility=global
  α/β - abc : Subsystem
  α/β - d/q : Subsystem
  PWM : Outport
  tag scope: P_deload_ref=global, idr=global, idr_ref=global, iqr=global, iqr_ref=global, theta_r=global
  wires:
  α/β - abc/1(Vabcr) -> 3er Harmonic Inyection/1(in)
  d/q - α/β/1(V αr/βr) -> α/β - abc/1(V αr/βr)
  iabcr/1 -> Gain 1 Trasnformer/1
  "abc - α/β "/1(i αr/βr) -> α/β - d/q/1(i αr/βr)
  3er Harmonic Inyection/1(out) -> Gain/1
  Theta_m (θm)/1 -> " Angle Rotor"/1(Theta_m (θm) Mechanic)
  Vabcs/1 -> " Angle Rotor"/2(Vabcs)
  " Angle Rotor"/1(theta_r (θr)) -> [theta_r], α/β - d/q/2(theta_r (θr))
  PI Id/1(Vd) -> Cancelation of cc/1(Vd)
  PI Iq/1(Vq) -> Cancelation of cc/2(Vq)
  α/β - d/q/1(i dr/qr) -> Demux/1
  Demux/2 -> [iqr]
  Demux/1 -> [idr]
  Q_ref/1 -> 1/kQ/1
  Cancelation of cc/1(Vdr  Vqr) -> d/q - α/β/1(Vdr  Vqr)
  Gain/1 -> Gain 2 Trasnformer/1
  Gain 1 Trasnformer/1 -> "abc - α/β "/1(iabcr)
  Gain 2 Trasnformer/1 -> PWM Generator (2-Level)/1
  PWM Generator (2-Level)/1 -> PWM/1
  1/kQ/1 -> [idr_ref], PI Id/1(idr_ref)
  Manual Switch/1 -> [iqr_ref], PI Iq/1(iqr_ref)
  [idr] -> PI Id/2(idr_means)
  [iqr] -> PI Iq/2(iqr_means)
  Constant2/1 -> Manual Switch5/1
  [f_dfig] -> Inertial Response1/1(f_means), Inertial Response/1(f_means), Display25/1, Deloaded Response/2(f_means)
  Manual Switch5/1 -> Display26/1, Deloaded Response/1(f_ref)
  [f_plant] -> Manual Switch5/2
  [theta_r] -> d/q - α/β/2(theta_r (θr))
  [omega_m] -> Zero-Order Hold3/1
  Zero-Order Hold3/1 -> Cancelation of cc/3(omega_m (Ωm))
  [P_dfig] -> Display24/1, P Control/2("Pot_means ")
  Sum1/1 -> Saturation1/1
  P Control/1(Id*_P) -> Manual Switch4/1, Display2/1
  1/kP1/1 -> Manual Switch4/2, Display1/1
  Manual Switch4/1 -> Display7/1, Manual Switch/2
  1/kT/1 -> Saturation/1
  P Control1/1(Id*_P) -> Display8/1, Manual Switch1/1
  Manual Switch1/1 -> Display3/1, Manual Switch/1
  Tem_ref/1 -> Display4/1, P Control1/1("T_ref "), 1/kT/1
  [Tem_mean] -> Display5/1, P Control1/2("T_means ")
  Saturation/1 -> Display6/1, Manual Switch1/2
  [Pot_ref_deload2] -> Manual Switch2/1
  iabc4/1 -> Manual Switch2/2
  Manual Switch2/1 -> Manual Switch6/2, Inertial Response1/2(P_deloaded)
  iabc6/1 -> Manual Switch3/2
  [Pot_max_ref2] -> Manual Switch3/1
  Manual Switch3/1 -> Inertial Response1/3(P_max)
  Saturation1/1 -> [P_deload_ref], Display22/1, P Control/1("Pot_ref "), 1/kP1/1
  Inertial Response1/1("P_deloaded ") -> Manual Switch6/1
  Deloaded Response/1("P_deloaded_dfig_ref ") -> Manual Switch7/2
  Manual Switch7/1 -> Sum1/1
  Constant1/1 -> Manual Switch7/1
  Constant3/1 -> Manual Switch8/1
  Inertial Response/1("Inertial_Res ") -> Manual Switch8/2
  Manual Switch8/1 -> Sum1/2
  Constant4/1 -> Manual Switch9/1
  Manual Switch6/1 -> Manual Switch9/2
  Manual Switch9/1 -> Sum1/3

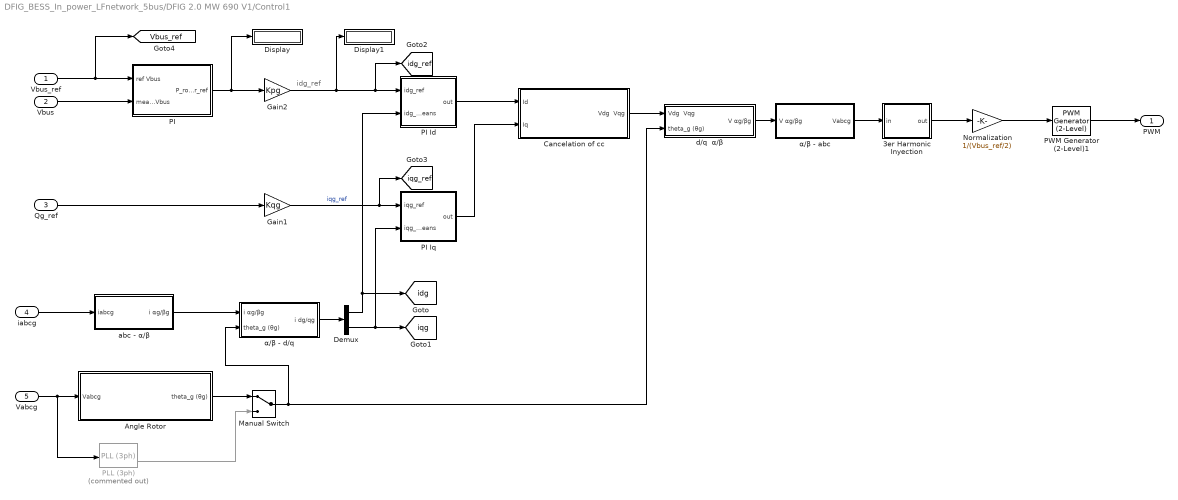
== system DFIG_BESS_In_power_LFnetwork_5bus/DFIG 2.0 MW 690 V1/Control1 ==
  note: idg_ref
  Vbus_ref : Inport
  Vbus : Inport  Port=2
  Qg_ref : Inport  Port=3
  iabcg : Inport  Port=4
  "Vabcg " : Inport  Port=5
  " Angle Rotor" : Subsystem
  3er Harmonic Inyection : Subsystem
  Cancelation of cc : Subsystem
  Demux : Demux  Outputs=2
  Display : Display
  Display1 : Display
  Gain1 : Gain  Gain=Kqg
  Gain2 : Gain  Gain=Kpg
  Manual Switch : ManualSwitch
  Normalization : Gain  Gain=1/(Vbus_ref/2)
  PI : Subsystem
  PI Id : Subsystem
  PI Iq : Subsystem
  PLL (3ph) : powerlib_meascontrol/PLL/PLL (3ph)  Commented=on  Fmin=45  Par_Init=[0, 60]  ParK=[180, 3200, 1]  TcD=1e-4  MaxRateChangeFreq=12  FilterCutOffFreq=25  Ts=0  AGC=on
      link override Model/abc to dq0: Alignment=Aligned with phase A axis
  PWM Generator (2-Level)1 : powerlib_meascontrol/Pulse & Signal Generators/PWM Generator (2-Level)  ModulatorType=Three-phase bridge (6 pulses)  ModulatorMode=Unsynchronized  Fc=fsw  Pc=0  nF=27  MinMax="[ -1  1 ]"  SamplingTechnique=Natural  ModulatingSignals=off  m=0.8  Freq=60  Phase=0  Ts=0  ShowCarrierOutport=off
      settings: SourceProductName=Simscape Power Systems
  "abc - α/β  " : Subsystem
  "d/q  α/β " : Subsystem
  α/β - abc : Subsystem
  α/β - d/q : Subsystem
  PWM : Outport
  tag scope: Vbus_ref=global, idg=global, idg_ref=global, iqg=global, iqg_ref=global
  wires:
  Normalization/1 -> PWM Generator (2-Level)1/1
  Cancelation of cc/1(Vdg  Vqg) -> "d/q  α/β "/1(Vdg  Vqg)
  Gain1/1 -> PI Iq/1(iqg_ref), [iqg_ref]  "iqg_ref"
  Demux/1 -> PI Id/2(idg_means), [idg]
  Demux/2 -> PI Iq/2(iqg_means), [iqg]
  PI Iq/1(out) -> Cancelation of cc/2(Iq)
  PI Id/1(out) -> Cancelation of cc/1(Id)
  3er Harmonic Inyection/1(out) -> Normalization/1
  "abc - α/β  "/1(i αg/βg) -> α/β - d/q/1(i αg/βg)
  "d/q  α/β "/1(V αg/βg) -> α/β - abc/1(V αg/βg)
  iabcg/1 -> "abc - α/β  "/1(iabcg)
  Vbus_ref/1 -> [Vbus_ref], PI/1("ref Vbus ")
  Gain2/1 -> Display1/1, [idg_ref], PI Id/1(idg_ref)
  Vbus/1 -> PI/2("means Vbus ")
  Qg_ref/1 -> Gain1/1
  α/β - abc/1(Vabcg) -> 3er Harmonic Inyection/1(in)
  "Vabcg "/1 -> " Angle Rotor"/1("Vabcg "), PLL (3ph)/1
  PI/1(P_rotor_ref) -> Display/1, Gain2/1
  " Angle Rotor"/1(theta_g (θg)) -> Manual Switch/1
  Manual Switch/1 -> "d/q  α/β "/2(theta_g (θg)), α/β - d/q/2(theta_g (θg))
  α/β - d/q/1(i dg/qg) -> Demux/1
  PLL (3ph)/2 -> Manual Switch/2
  PWM Generator (2-Level)1/1 -> PWM/1

== system DFIG_BESS_In_power_LFnetwork_5bus/DFIG 2.0 MW 690 V1/Deload method 1 ==
  Wind speed (m/s) : Inport
  CP : Constant  Value=0.40
  CP1 : Constant  Value=0.44
  Display1 : Display
  Display2 : Display
  Mux6 : Mux  Inputs=2
  Mux7 : Mux  Inputs=2
  Pt_deload : Fcn  Expr=0.5*ro*pi*(Radio)^2*(u[1])^3*u[2]
  Pt_max : Fcn  Expr=0.5*ro*pi*(Radio)^2*(u[1])^3*u[2]
  Scope1 : Scope  NumInputPorts=2
  Sum : Sum  Inputs=|-+
  P_deload : Outport
  P_Max : Outport  Port=2
  P_backup : Outport  Port=3
  wires:
  CP/1 -> Mux6/2
  Mux6/1 -> Pt_deload/1
  Wind speed (m/s)/1 -> Mux7/1, Mux6/1
  Mux7/1 -> Pt_max/1
  CP1/1 -> Mux7/2
  Pt_deload/1 -> Sum/1, Display2/1, Scope1/1, P_deload/1
  Pt_max/1 -> Sum/2, P_Max/1, Display1/1, Scope1/2
  Sum/1 -> P_backup/1

== system DFIG_BESS_In_power_LFnetwork_5bus/DFIG 2.0 MW 690 V1/MPPT & Deload method 2 ==
  note: Zone 2: MPPT with Vw 5 - 11
  Omega_m : Inport
  Deloaded : Gain  Gain=0.88
  Display{1..4} (4 alike) : Display
  Gearbox Ratio Generator Torque (-)1 : Gain  Gain=-1/N
  Gearbox Ratio1 : Gain  Gain=1/N
  Kopt : Gain  Gain=0.5*ro*pi*(Radio)^5/(lambda_opt)^3*cp_opt_abs
  Product2 : Product  Inputs=**  SaturateOnIntegerOverflow=on  InputSameDT=on  OutDataTypeStr=Inherit: Same as first input
  Saturation : Saturate  UpperLimit=2.5e+06  LowerLimit=0
  omega^2 : Fcn  Expr=(u[1])^2
  Tem_ref : Outport
  "Pot_max_ref " : Outport  Port=2
  "Pot_ref_deload2 " : Outport  Port=3
  wires:
  Gearbox Ratio1/1 -> Product2/2, omega^2/1
  omega^2/1 -> Kopt/1
  Kopt/1 -> Product2/1, Display3/1, Gearbox Ratio Generator Torque (-)1/1
  Product2/1 -> Saturation/1  "Pt"
  Gearbox Ratio Generator Torque (-)1/1 -> Display2/1, Tem_ref/1
  Omega_m/1 -> Gearbox Ratio1/1
  Saturation/1 -> Deloaded/1, Display1/1, "Pot_max_ref "/1
  Deloaded/1 -> Display4/1, "Pot_ref_deload2 "/1

== system DFIG_BESS_In_power_LFnetwork_5bus/DFIG 2.0 MW 690 V1/Measurement of Power - Frequency ==
  FP : Fcn  Commented=on  Expr=cos(atan(u[1]/u[2]))
  Manual Switch3 : ManualSwitch
  Mux : Mux  Commented=on  Inputs=2
  PLL (3ph)1 : powerlib_meascontrol/PLL/PLL (3ph)  Commented=on  Fmin=45  Par_Init=[0, f]  ParK=[180, 3200, 1]  TcD=1e-4  MaxRateChangeFreq=12  FilterCutOffFreq=25  Ts=0  AGC=on
  "Power (3ph, Instantaneous)1" : powerlib_meascontrol/Measurements/Power (3ph, Instantaneous)
      settings: SourceProductName=Simscape Power Systems
  Scope : Scope  Commented=on
  F (Hz) : Outport
  P (W) : Outport  Port=2
  Q (VAR) : Outport  Port=3
  Angle (0) : Outport  Port=4
  tag scope: P_dfig=global, Q_dfig=global, f_dfig=global, wt_mean_dfig=global
  wires:
  [Vdfig] -> "Power (3ph, Instantaneous)1"/1, PLL (3ph)1/1
  "Power (3ph, Instantaneous)1"/1 -> Mux/2, P (W)/1, [P_dfig]  "Pot"
  [Idfig] -> "Power (3ph, Instantaneous)1"/2
  "Power (3ph, Instantaneous)1"/2 -> Mux/1, Q (VAR)/1, [Q_dfig]
  PLL (3ph)1/2 -> Angle (0)/1, [wt_mean_dfig]
  Mux/1 -> FP/1
  FP/1 -> Scope/1
  [f_dfig_bess] -> Manual Switch3/1
  Manual Switch3/1 -> [f_dfig], F (Hz)/1
  PLL (3ph)1/1 -> Manual Switch3/2

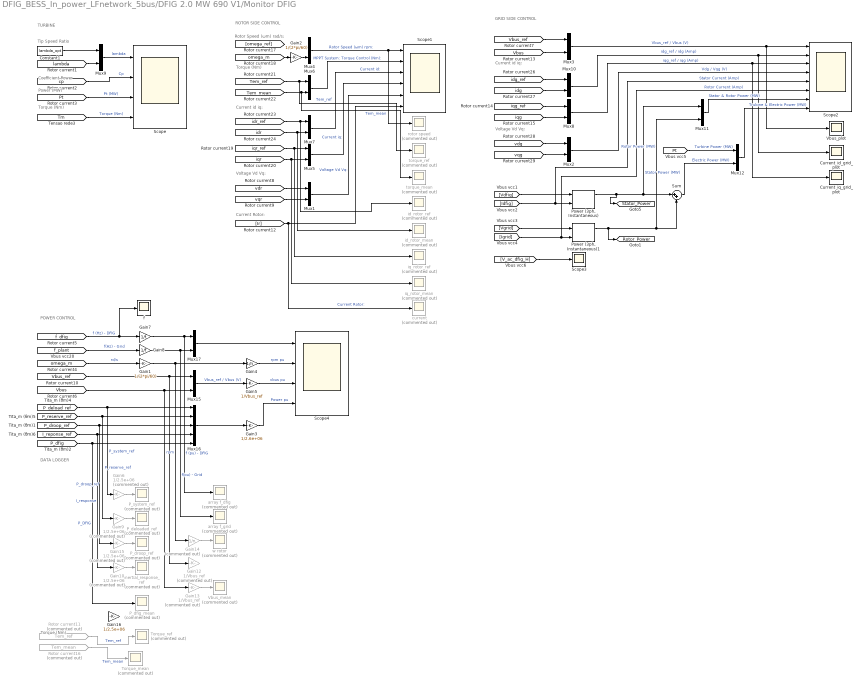
== system DFIG_BESS_In_power_LFnetwork_5bus/DFIG 2.0 MW 690 V1/Monitor DFIG ==
  note: ROTOR SIDE CONTROL
  note: Torque (Nm)
  note: Current id iq:
  note: Rotor Speed (ωm) rad/s:
  note: Voltage Vd Vq:
  note: TURBINE
  note: Torque (Nm)
  note: Power (MW)
  note: Coefficient Power
  note: Tip Speed Ratio
  note: GRID SIDE CONTROL
  note: Current id iq:
  note: Voltage Vd Vq:
  note: Current Rotor:
  note: POWER CONTROL
  note: DATA LOGGER
  note: Torque (Nm)
  Constant1 : Constant  Value=lambda_opt
  Current_id_grid_plot : Scope
  Current_iq_grid_plot : Scope
  Gain1 : Gain  Gain=1/(2*pi/60)
  Gain{6,9..10,15} (4 alike) : Gain  Commented=on  Gain=1/2.5e+06
  Gain12 : Gain  Commented=on  Gain=1/Vbus_ref
  Gain13 : Gain  Commented=on  Gain=1/Vbus_ref
  Gain14 : Gain  Commented=on  Gain=1/n
  Gain16 : Gain  Gain=1/2.5e+06
  Gain2 : Gain  Gain=1/(2*pi/60)
  Gain3 : Gain  Gain=1/2.6e+06
  Gain4 : Gain  Gain=1/n
  Gain5 : Gain  Gain=1/Vbus_ref
  Gain7 : Gain  Gain=1/f
  Gain8 : Gain  Gain=1/f
  Inertial_response_ref : Scope  Commented=on
  Mux{1..12,15,17} (14 alike) : Mux  Inputs=2
  Mux16 : Mux  Inputs=5
  P_deloaded_ref : Scope  Commented=on
  P_dfig_mean : Scope  Commented=on
  P_droop_ref : Scope  Commented=on
  P_system_ref : Scope  Commented=on
  "Power (3ph, Instantaneous)" : powerlib_meascontrol/Measurements/Power (3ph, Instantaneous)
      settings: SourceProductName=Simscape Power Systems
  "Power (3ph, Instantaneous)1" : powerlib_meascontrol/Measurements/Power (3ph, Instantaneous)
      settings: SourceProductName=Simscape Power Systems
  Rotor current11 : From  Commented=on  GotoTag=Tem_ref  TagVisibility=global
  Rotor current16 : From  Commented=on  GotoTag=Tem_mean  TagVisibility=global
  Scope : Scope  NumInputPorts=4
  Scope1 : Scope  NumInputPorts=6
  Scope2 : Scope  NumInputPorts=8
  Scope3 : Scope
  Scope4 : Scope  NumInputPorts=4
  Sum : Sum  Inputs=|++
  Torque_mean : Scope  Commented=on
  Torque_ref : Scope  Commented=on
  Vbus_mean : Scope  Commented=on
  Vbus_plot : Scope
  array f_dfig : Scope  Commented=on
  array f_grid : Scope  Commented=on
  current : Scope  Commented=on
  f : Scope
  id_rotor_mean : Scope  Commented=on
  id_rotor_ref : Scope  Commented=on
  iq_rotor_mean : Scope  Commented=on
  iq_rotor_ref : Scope  Commented=on
  rotor speed : Scope  Commented=on
  torque_mean : Scope  Commented=on
  torque_ref : Scope  Commented=on
  w rotor : Scope  Commented=on
  tag scope: Rotor_Power=global, Stator_Power=global
  wires:
  [iqr_ref] -> iq_rotor_ref/1, Mux5/1
  [iqr] -> iq_rotor_mean/1, Mux5/2
  [idr] -> id_rotor_mean/1, Mux7/2
  [idr_ref] -> id_rotor_ref/1, Mux7/1
  [vdr] -> Mux1/1
  [vqr] -> Mux1/2
  [vqg] -> Mux2/2
  [vdg] -> Mux2/1
  [idg_ref] -> Mux10/1
  [idg] -> Mux10/2
  [iqg] -> Mux8/2
  [iqg_ref] -> Mux8/1
  [Tem_ref] -> torque_ref/1, Mux6/1  "Tem_ref"
  [Vbus] -> Mux3/2
  [Vbus_ref] -> Mux3/1
  [cp] -> Scope/2  "Cp"
  [Pt] -> Scope/3  "Pt (MW)"
  [Tm] -> Scope/4  "Torque (Nm)"
  Mux4/1 -> rotor speed/1, Scope1/1  "Rotor Speed (ωm) rpm:"
  Mux6/1 -> Scope1/2  "MPPT System: Torque Control (Nm):"
  Mux7/1 -> Scope1/3  "Current id:"
  Mux5/1 -> Scope1/4  "Current iq:"
  Mux1/1 -> Scope1/5  "Voltage Vd Vq:"
  [Ir] -> current/1, Scope1/6  "Current Rotor:"
  [omega_m] -> Gain2/1
  Gain2/1 -> Mux4/2
  Mux3/1 -> Vbus_plot/1, Scope2/1  "Vbus_ref / Vbus (V)"
  Mux10/1 -> Current_id_grid_plot/1, Scope2/2  "idg_ref / idg (Amp)"
  Mux8/1 -> Scope2/3, Current_iq_grid_plot/1  "iqg_ref / iqg (Amp)"
  Mux2/1 -> Scope2/4  "Vdg / Vqg (V)"
  [lambda] -> Mux9/2
  Constant1/1 -> Mux9/1
  Mux9/1 -> Scope/1  "lambda"
  [Tem_mean] -> torque_mean/1, Mux6/2  "Tem_mean"
  [Vdfig] -> "Power (3ph, Instantaneous)"/1
  [Vgrid] -> "Power (3ph, Instantaneous)1"/1
  [Igrid] -> "Power (3ph, Instantaneous)1"/2, Scope2/6  "Rotor Current (Amp)"
  [Idfig] -> "Power (3ph, Instantaneous)"/2, Scope2/5  "Stator Current (Amp)"
  "Power (3ph, Instantaneous)"/1 -> [Stator_Power], Mux11/1, Sum/1  "Stator Power (MW)"
  "Power (3ph, Instantaneous)1"/1 -> [Rotor_Power], Sum/2, Mux11/2  "Rotor Power (MW)"
  Sum/1 -> Mux12/2  "Electric Power (MW)"
  Mux11/1 -> Scope2/7  "Stator & Rotor Power (MW)"
  [Pt] -> Mux12/1  "Turbine Power (MW)"
  Mux12/1 -> Scope2/8  "Trubine & Electric Power (MW)"
  [V_ac_dfig_H] -> Scope3/1
  [omega_m] -> Gain1/1  "rd/s"
  [Vbus] -> Gain13/1, Mux15/2
  [Vbus_ref] -> Gain12/1, Mux15/1
  [P_deload_ref] -> Gain6/1, Mux16/1  "P_system_ref"
  [P_reserve_ref] -> Gain9/1, Mux16/2  "P_reserve_ref"
  [I_reponse_ref] -> Mux16/4, Gain10/1  "I_response"
  Mux17/1 -> Scope4/1
  [f_dfig] -> f/1, Gain7/1  "f (Hz) - DFIG"
  [f_plant] -> Gain8/1  "f(Hz) - Grid"
  Gain1/1 -> Gain14/1, Gain4/1  "rpm"
  Mux15/1 -> Gain5/1  "Vbus_ref / Vbus (V)"
  [P_dfig] -> P_dfig_mean/1, Mux16/5  "P_DFIG"
  Gain4/1 -> Scope4/2  "rpm pu"
  Gain5/1 -> Scope4/3  "vbus pu"
  Mux16/1 -> Gain3/1
  Gain7/1 -> array f_dfig/1, Mux17/1  "f (pu) - DFIG"
  Gain8/1 -> array f_grid/1, Mux17/2  "f(pu) - Grid"
  Gain3/1 -> Scope4/4  "Power pu"
  Gain6/1 -> P_system_ref/1
  Gain9/1 -> P_deloaded_ref/1
  Gain10/1 -> Inertial_response_ref/1
  Gain13/1 -> Vbus_mean/1
  Gain14/1 -> w rotor/1
  [P_droop_ref] -> Gain15/1, Mux16/3  "P_droop_ref"
  Gain15/1 -> P_droop_ref/1
  Rotor current11/1 -> Torque_ref/1  "Tem_ref"
  Rotor current16/1 -> Torque_mean/1  "Tem_mean"

== system DFIG_BESS_In_power_LFnetwork_5bus/DFIG 2.0 MW 690 V1/Signal Builder ==
  Demux : Demux  Tag=STV Demux  Outputs=1
  FromWs : FromWorkspace  Tag=STV FromWs  VariableName=tuvar  SampleTime=0
      SigBuilderData=|
      | common.afterFinalStr = 'Extrapolate'
      | common.sampleTime = 0
      | dataSet.timeRange = [0 20]
      | dataSet.name = 'Group 1'
      | sbobj.Groups.Name = 'Group 1'
      | sbobj.Groups.Signals.Name = 'Signal 1'
      | sbobj.Groups.Signals.XData = [0 1.5 4.8 5 5.2 5.44 5.7 6.08 6.5 6.84 7.18 7.62 8 8.42 8.98 9.48 10 10.4 10.88 11.36 11.8 12.32 12.88 13.38 14.1 14.74 15.28 15.86 16.32 16.86 17.5 18.1 18.62 19.32 20]
      | sbobj.Groups.Signals.YData = [0 11.5 11.5471428571 11.4 10.3 9.95 9.75 10.05 10.5 10.95 11.1 11.15 11.55 11.65 11.5 11.3 11.35 11.35 11.45 11.35 11.15 11.35 11.5 11.4859550562 11.55 11.5228813559 11.5 11.4754237288 11.4559322034 11.4330508475 11.4059322034 11.3805084746 11.3584745763 11.3288135593 11.3]
      | sbobj.Groups.TimeRange = [0 20]
  Signal 1 : Outport  Tag=STV Outport
  wires:
  Demux/1 -> Signal 1/1
  FromWs/1 -> Demux/1

== system DFIG_BESS_In_power_LFnetwork_5bus/DFIG 2.0 MW 690 V1/Subsystem ==
  In1 : Inport
  Bus Selector : BusSelector  OutputSignals=Mechanical.Rotor angle thetam (rad),Mechanical.Rotor speed (wm),Mechanical.Electromagnetic torque Te (N*m)
  tag scope: Tem_mean=global, omega_m=global, tita_m=global
  wires:
  Bus Selector/2 -> [omega_m]  "<Rotor speed (wm)>"
  In1/1 -> Bus Selector/1
  Bus Selector/1 -> [tita_m]  "<Rotor angle thetam (rad)>"
  Bus Selector/3 -> [Tem_mean]  "<Electromagnetic torque Te (N*m)>"
